simulink model "case_10_lead_car_steady_ego_car_steady"  (R2025a)
settings: Solver=VariableStepAuto  StartTime=0.0  StopTime=20  RelTol=1e-3
settings Model: Creator=sanborkl  LastModifiedBy=sanborkl

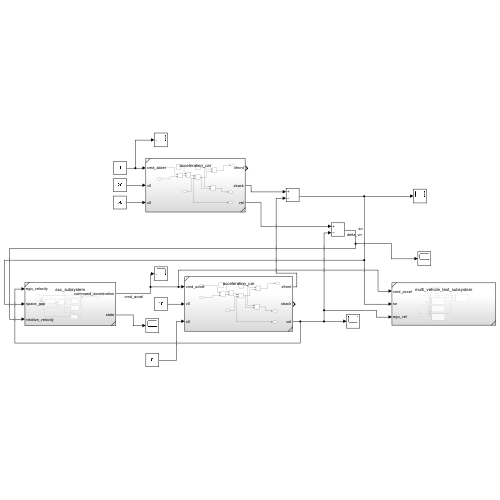
[thumbnail: Simulink's stored preview of the top-level diagram]
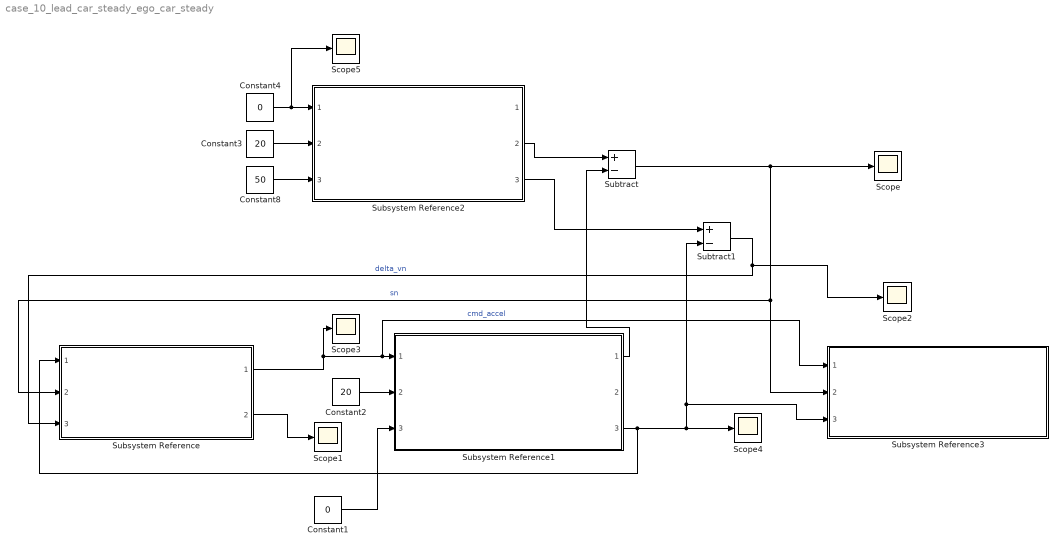
== system case_10_lead_car_steady_ego_car_steady ==
  Constant1 : Constant  Value=0
  Constant2 : Constant  Value=20
  Constant3 : Constant  Value=20
  Constant4 : Constant  Value=0
  Constant8 : Constant  Value=50
  Scope{,1..5} (6 alike) : Scope
      Scope settings: ActiveDisplayYMinimum=39.280054202245637  ActiveDisplayYMaximum=46.479993977528267
      Scope1 settings: ActiveDisplayYMinimum=-1  ActiveDisplayYMaximum=1  DataLoggingVariableName=ScopeData2
      Scope2 settings: ActiveDisplayYMinimum=-2.4298440672339487  ActiveDisplayYMaximum=0.26998267413710536  DataLoggingVariableName=ScopeData3
      Scope3 settings: ActiveDisplayYMinimum=-1.6601447210305178  ActiveDisplayYMaximum=1.8511271912256131  DataLoggingVariableName=ScopeData4
      Scope4 settings: ActiveDisplayYMinimum=-1  ActiveDisplayYMaximum=1
      Scope5 settings: ActiveDisplayYMinimum=-1.75  ActiveDisplayYMaximum=5.75  DataLoggingVariableName=ScopeData5
  Subsystem Reference : Subsystem  ReferencedSubsystem=acc_subsystem
  Subsystem Reference1 : Subsystem  ReferencedSubsystem=acceleration_car
  Subsystem Reference2 : Subsystem  ReferencedSubsystem=acceleration_car
  Subsystem Reference3 : Subsystem  ReferencedSubsystem=multi_vehicle_test_subsystem
  Subtract : Sum  Inputs=+-
  Subtract1 : Sum  Inputs=+-
  wires:
  Subsystem Reference2/3 -> Subtract1/1
  Constant3/1 -> Subsystem Reference2/2
  Constant2/1 -> Subsystem Reference1/2
  Subsystem Reference1/1 -> Subtract/2
  Subsystem Reference/1 -> Scope3/1, Subsystem Reference3/1, Subsystem Reference1/1  "cmd_accel"
  Constant1/1 -> Subsystem Reference1/3
  Subsystem Reference/2 -> Scope1/1
  Subsystem Reference2/2 -> Subtract/1
  Subtract/1 -> Subsystem Reference3/2, Subsystem Reference/2, Scope/1  "sn"
  Subsystem Reference1/3 -> Subsystem Reference/1, Subtract1/2, Subsystem Reference3/3, Scope4/1
  Subtract1/1 -> Scope2/1, Subsystem Reference/3  "delta_vn"
  Constant8/1 -> Subsystem Reference2/3
  Constant4/1 -> Scope5/1, Subsystem Reference2/1
